simulink model "quest2_2"  (R2015b)
settings: Solver=ode45  StartTime=0.0  StopTime=2  FixedStep=0.001  RelTol=1e-3
values from neighbouring files (symbols this model uses):
  Kpx = 5    [staticInit.m]
  Kpy = 5    [staticInit.m]
  L = 0.13    [staticInit.m]
  r = 0.1    [staticInit.m]
  Xfinal = -4    [staticInit.m]
  Yfinal = 4    [staticInit.m]
undefined symbols (not defined in the file or in its folder): F_invW
libraries: simulink x1
settings Model: Creator=Subodh  LastModifiedBy=Subodh
settings HardwareCC: ProdWordSize=32  ProdHWDeviceType=Specified

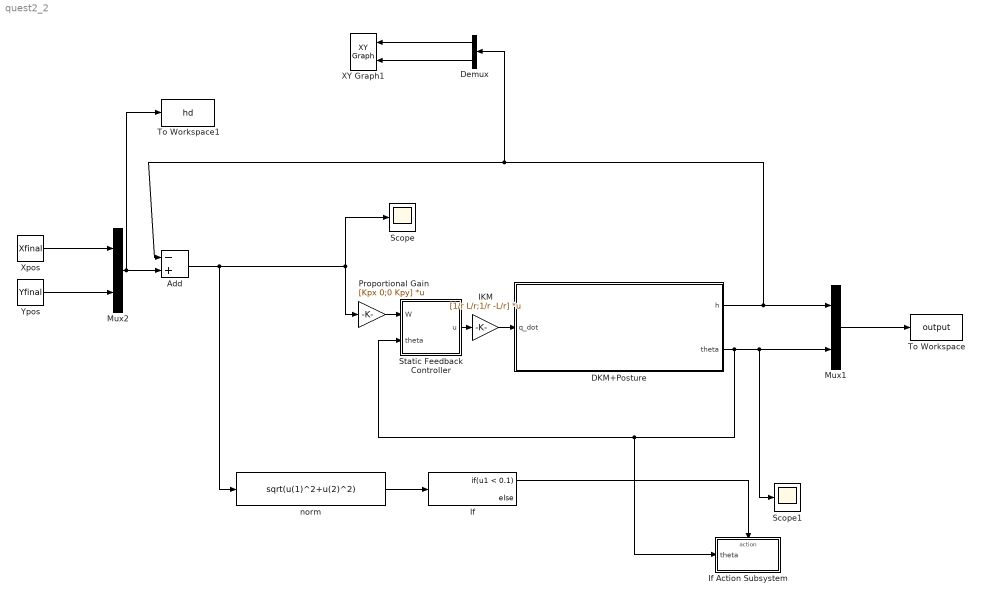
== system quest2_2 ==
  Add : Sum  Inputs=-+
  DKM+Posture : Subsystem
  Demux : Demux  Outputs=2
  IKM : Gain  Gain=[1/r L/r;1/r -L/r]  Multiplication=Matrix(K*u)
  If : If  IfExpression=u1 < 0.1
  If Action Subsystem : Subsystem  TreatAsAtomicUnit=on
  Mux1 : Mux  Inputs=2
  Mux2 : Mux  Inputs=2
  Proportional Gain : Gain  Gain=[Kpx 0;0 Kpy]  Multiplication=Matrix(K*u)
  Scope : Scope
  Scope1 : Scope
  Static Feedback Controller : Subsystem
  To Workspace : ToWorkspace  VariableName=output  SampleTime=-1
  To Workspace1 : ToWorkspace  VariableName=hd  SampleTime=-1
  XY Graph1 : simulink/Sinks/XY Graph  xmin=-2.5  xmax=2.5  ymin=-2.5  ymax=2.5  st=-1
  Xpos : Constant  Value=Xfinal
  Ypos : Constant  Value=Yfinal
  norm : Fcn  Expr=sqrt(u(1)^2+u(2)^2)
  wires:
  Mux1/1 -> To Workspace/1
  Add/1 -> norm/1, Scope/1, Proportional Gain/1
  Mux2/1 -> Add/2, To Workspace1/1
  Xpos/1 -> Mux2/1
  Static Feedback Controller/1(u) -> IKM/1
  DKM+Posture/2(theta) -> Scope1/1, Mux1/2, If Action Subsystem/1(theta), Static Feedback Controller/2(theta)
  Demux/2 -> XY Graph1/2
  Proportional Gain/1 -> Static Feedback Controller/1(W)
  DKM+Posture/1(h) -> Demux/1, Add/1, Mux1/1
  Demux/1 -> XY Graph1/1
  IKM/1 -> DKM+Posture/1(q_dot)
  Ypos/1 -> Mux2/2
  norm/1 -> If/1
  If/1 -> If Action Subsystem/Action

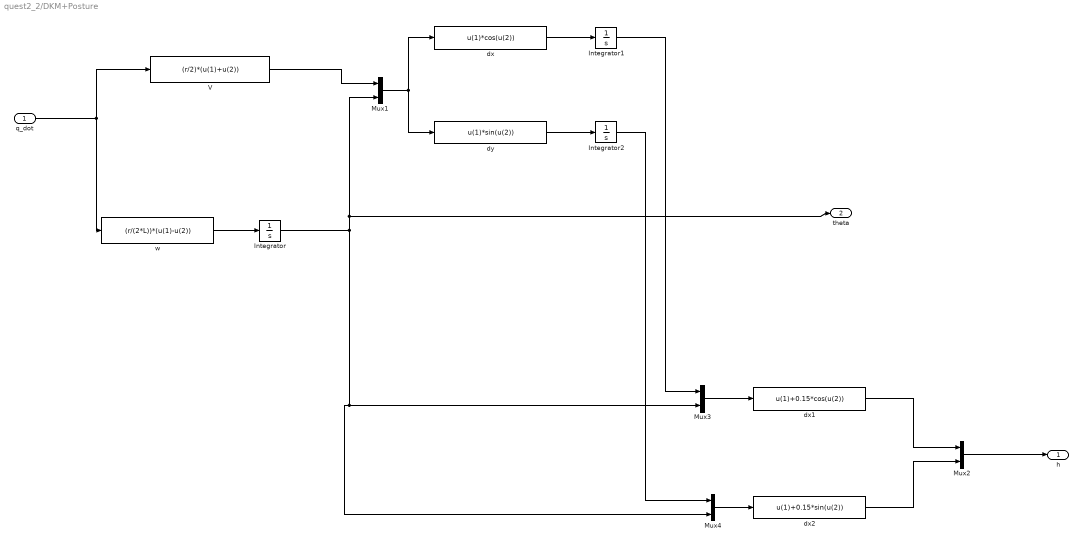
== system quest2_2/DKM+Posture ==
  q_dot : Inport
  Integrator : Integrator  InitialCondition=pi
  Integrator1 : Integrator  InitialCondition=2.45
  Integrator2 : Integrator
  Mux{1..4} (4 alike) : Mux  Inputs=2
  V : Fcn  Expr=(r/2)*(u(1)+u(2))
  dx : Fcn  Expr=u(1)*cos(u(2))
  dx1 : Fcn  Expr=u(1)+0.15*cos(u(2))
  dx2 : Fcn  Expr=u(1)+0.15*sin(u(2))
  dy : Fcn  Expr=u(1)*sin(u(2))
  w : Fcn  Expr=(r/(2*L))*(u(1)-u(2))
  h : Outport
  theta : Outport  Port=2
  wires:
  q_dot/1 -> V/1, w/1
  w/1 -> Integrator/1
  Integrator1/1 -> Mux3/1
  dy/1 -> Integrator2/1
  Mux1/1 -> dy/1, dx/1
  Integrator2/1 -> Mux4/1
  dx/1 -> Integrator1/1
  V/1 -> Mux1/1
  Integrator/1 -> Mux4/2, Mux3/2, Mux1/2, theta/1
  Mux2/1 -> h/1
  Mux3/1 -> dx1/1
  Mux4/1 -> dx2/1
  dx1/1 -> Mux2/1
  dx2/1 -> Mux2/2

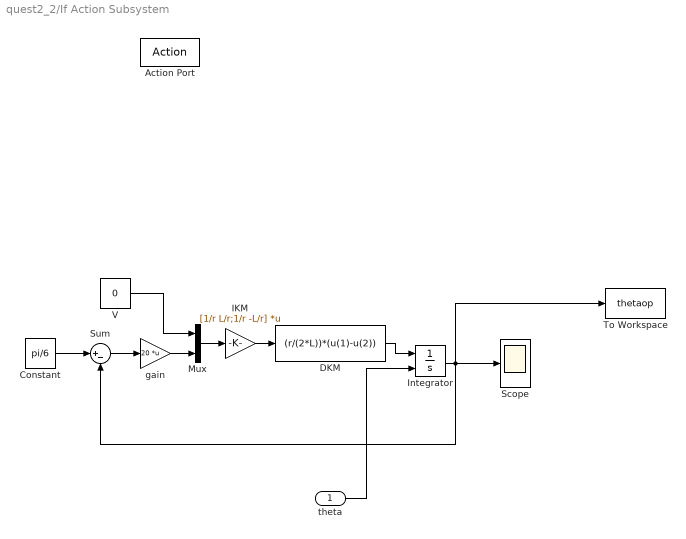
== system quest2_2/If Action Subsystem ==
  theta : Inport
  Action Port : ActionPort  ActionType=then
  Constant : Constant  Value=pi/6
  DKM : Fcn  Expr=(r/(2*L))*(u(1)-u(2))
  IKM : Gain  Gain=[1/r L/r;1/r -L/r]  Multiplication=Matrix(K*u)
  Integrator : Integrator  InitialConditionSource=external
  Mux : Mux  Inputs=2
  Scope : Scope
  Sum : Sum  Inputs=|+-
  To Workspace : ToWorkspace  VariableName=thetaop  SampleTime=-1
  V : Constant  Value=0
  gain : Gain  Gain=20  Multiplication=Matrix(K*u)
  wires:
  Constant/1 -> Sum/1
  Integrator/1 -> To Workspace/1, Scope/1, Sum/2
  theta/1 -> Integrator/2
  Sum/1 -> gain/1
  gain/1 -> Mux/2
  Mux/1 -> IKM/1
  IKM/1 -> DKM/1
  DKM/1 -> Integrator/1
  V/1 -> Mux/1

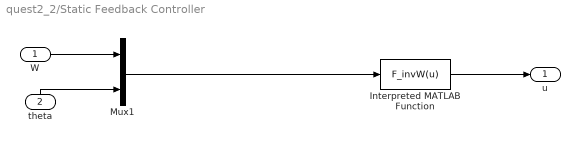
== system quest2_2/Static Feedback Controller ==
  W : Inport
  theta : Inport  Port=2
  Interpreted MATLAB Function : MATLABFcn  MATLABFcn=F_invW(u)  OutputSignalType=real  Output1D=off
  Mux1 : Mux  Inputs=2
  u : Outport
  wires:
  theta/1 -> Mux1/2
  W/1 -> Mux1/1
  Interpreted MATLAB Function/1 -> u/1
  Mux1/1 -> Interpreted MATLAB Function/1
